simulink model "Crouzet_DC_motor"  (R2020a)
settings: Solver=VariableStepAuto  StartTime=0.0  StopTime=10.0  RelTol=1e-3  EnableMultiTasking=on
settings Model: Creator=admin_aboyer  LastModifiedBy=admin_aboyer
settings DataIOCC: ReturnWorkspaceOutputs=off
settings OptimizationCC: LifeSpan=inf
settings DebuggingCC: SFUnexpectedBacktrackingDiag=warning  SFNoUnconditionalDefaultTransitionDiag=warning  ArithmeticOperatorsInVariantConditions=warning
settings SFSimCC: SimUseLocalCustomCode=off  CustomCodeUndefinedFunction=UseInterfaceOnly
settings RTWCC: RTWUseLocalCustomCode=off
settings CodeAppCC: StateflowObjectComments=on
settings GRTTargetCC: TargetLangStandard=C89/C90 (ANSI)
settings ConfigComp: CovMetricSettings=dw  CovHtmlReporting=on  CovSaveCumulativeToWorkspaceVar=on  CovSaveSingleToWorkspaceVar=on  CovExternalEMLEnable=off

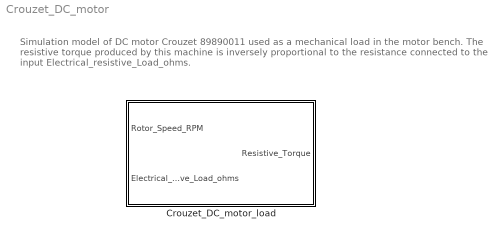
== system Crouzet_DC_motor ==
  note: Simulation model of DC motor Crouzet 89890011 used as a mechanical load in the motor bench.
      | The resistive torque produced by this machine is inversely proportional to the resistance
      | connected to the input Electrical_resistive_Load_ohms.
  Crouzet_DC_motor_load : Subsystem

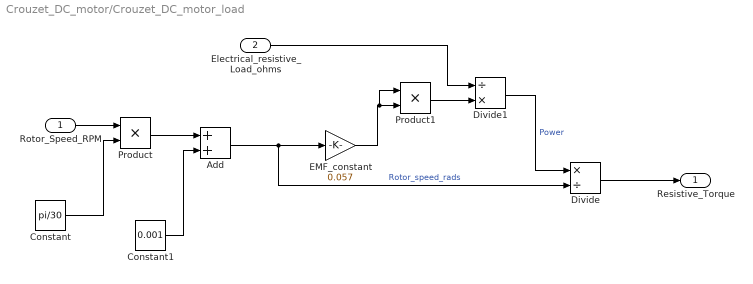
== system Crouzet_DC_motor/Crouzet_DC_motor_load ==
  Rotor_Speed_RPM : Inport
  Electrical_resistive_Load_ohms : Inport  Port=2
  Add : Sum
  Constant : Constant  Value=pi/30
  Constant1 : Constant  Value=0.001
  Divide : Product  Inputs=*/
  Divide1 : Product  Inputs=/*
  EMF_constant : Gain  Gain=0.057
  Product : Product
  Product1 : Product
  Resistive_Torque : Outport
  wires:
  Rotor_Speed_RPM/1 -> Product/1
  Constant/1 -> Product/2
  Product/1 -> Add/1
  Constant1/1 -> Add/2
  Add/1 -> Divide/2, EMF_constant/1  "Rotor_speed_rads"
  EMF_constant/1 -> Product1/1, Product1/2
  Product1/1 -> Divide1/2
  Divide1/1 -> Divide/1  "Power"
  Divide/1 -> Resistive_Torque/1
  Electrical_resistive_Load_ohms/1 -> Divide1/1
